simulink library "csf"  (Simulink 8.1)
settings: Solver=ode1  StartTime=0.0  StopTime=Inf  FixedStep=0.001  RelTol=1e-3
PostLoadFcn:
  | , if any(exist('dsrtsu_mdlpostloadfcn', 'file') == [2, 3, 6]), try dsrtsu_mdlpostloadfcn('Execute', bdroot); catch fprintf('Error in PostLoadFcn (dsrtsu_mdlpostloadfcn) for model "%s":\n %s\n', bdroot, lasterr); end, end,
undefined symbols (not defined in the file or in its folder): C_TICK_TIME_S, KJUD_VSCalcRollAvgInterval_s
libraries: hcu_lib x1
settings Model: DSRTSU_INTERNAL_RTI_VER=450  DSRTSU_INTERNAL_RTI_TYPE=rti1401  RTICANMMDATA=struct('GeneralSetupData',struct('modelroot','D:\ELN150201_TAIWAN\trunk\AdasDragon\software\sw_development\arch\app\jud','generalsettings',struct('filesettings',struct('destfolder',struct('Name','RTICANMM_FILES','Check',1),'buildfolder',struct('Name','.','Check',1),'AbsDestfolder',struct('Name','D:\ELN150201_TAIWAN\trunk\AdasDragon\software\sw_development\arch\app\jud\RTICANMM_FILES'),'AbsBuildfolder',struct('Name','D:\ELN150201_TAIWAN\trunk\AdasDragon\software\sw_development\arch\app\jud'))),'options',struct('addpaths',1,'rmpaths',1,'addtrcexclusion',logical(1),'cannavigator',struct('checkmonitoring',0),'show_usrtrc',0,'use_usrtrc',0),'advanced',struct('options',[1 1 1 1 1 1 1 1 1 1 1 1 1 1 1 1 1 1 1 1 1 1 1 1 1 1 1 1 1 1 1 1 1 1 1 1 1 1 1 1 1 1 1 1 1 1 1 1 1 1 1 1 1 1 1 1 1 1 1 1 1 1 1 1 1 1 1 1 1 1 1 1 1 1 1 1 1 1 1 1 1 1 1 1 1 1 1 1 1 1 1 1 1 1 1 1 1 1 1 1]),'MPSetup',{{}},'modelname','csf','block','csf'))  DSRTSU_INTERNAL_RTIFPGA=40  Creator=AT015555  LastModifiedBy=AT015555

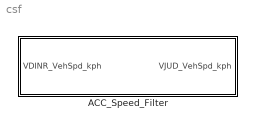
== system csf ==
  ACC_Speed_Filter : Subsystem

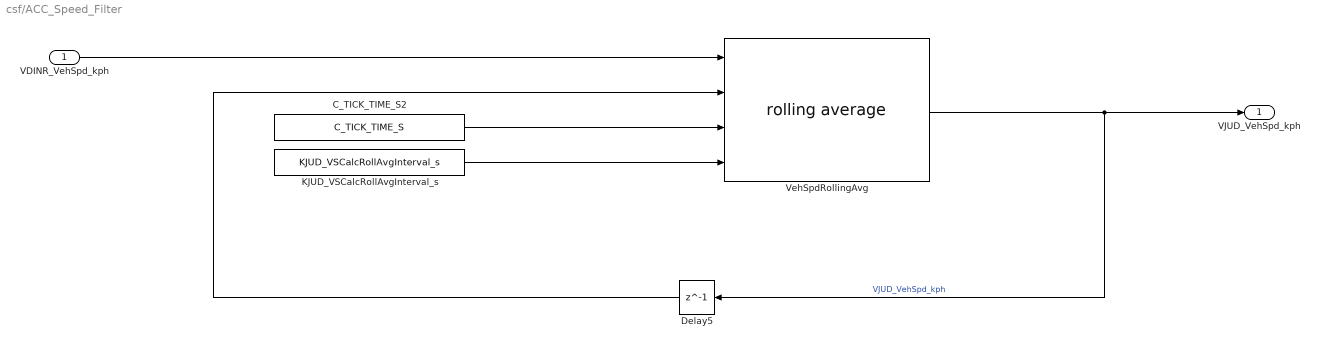
== system csf/ACC_Speed_Filter ==
  VDINR_VehSpd_kph : Inport
  C_TICK_TIME_S2 : Constant  Value=C_TICK_TIME_S
  Delay5 : Delay  DelayLength=1
  KJUD_VSCalcRollAvgInterval_s : Constant  Value=KJUD_VSCalcRollAvgInterval_s
  VehSpdRollingAvg : hcu_lib/rolling average
  VJUD_VehSpd_kph : Outport
  wires:
  C_TICK_TIME_S2/1 -> VehSpdRollingAvg/3
  KJUD_VSCalcRollAvgInterval_s/1 -> VehSpdRollingAvg/4
  Delay5/1 -> VehSpdRollingAvg/2
  VDINR_VehSpd_kph/1 -> VehSpdRollingAvg/1
  VehSpdRollingAvg/1 -> Delay5/1, VJUD_VehSpd_kph/1  "VJUD_VehSpd_kph"
